simulink library "powerlib11"  (Simulink 6.0)
settings: Solver=ode45  SolverMode=SingleTasking  StartTime=0.0  StopTime=10.0  RelTol=1e-3
libraries: powerlib2 x45
settings Model: Creator=barnard  LastModifiedBy=batserve  ExtModeAutoUpdateStatusClock=off
settings OptimizationCC: BooleanDataType=off
settings DebuggingCC: SolverPrmCheckMsg=none
settings HardwareCC: TargetUnknown=on

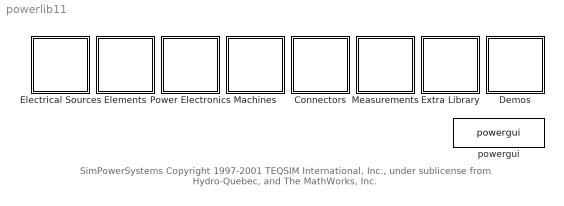
== system powerlib11 ==
  note: SimPowerSystems
      | Copyright  1997-2001 TEQSIM International, Inc., under sublicense
      | from Hydro-Quebec, and The MathWorks, Inc.
  Connectors : Subsystem
      mask Display: plot(0,0,100,100,[80,40],[40,40],[70,51],[31,31],[64,57],[23,23],[5,60,60],[70,70,40],[32,32],[70,97],[31,32,34,29,29,34,34,29,34,29],[71,68,71,71,70,68,71,68,68,71])
  Demos : Subsystem
      settings: OpenFcn=demo('simulink','SimPowerSystems')
      mask Display: disp('Demos')
  Electrical Sources : Subsystem
      mask Display: plot(-15,-15,15,15,[0 0 5 -5],[10 1.25 1.25 1.25],[0 0 -2 2],[-10 -1.25 -1.25 -1.25],[6 4 5 5 5]-10,[3 3 3 4 2]+3)
  Elements : Subsystem
      mask Display: plot(0,0,100,100,[90,64,77,77,60,56,51,46,40,34,30,25,13],[57,57,57,80,80,65,94,65,94,65,94,80,80],[90,87,82,77,74,68,64],[43,46,48,48,48,46,43],[48,77,77],[20,20,48],[39,27,13],[36,20,20])
  Extra Library : Subsystem
      settings: OpenFcn=powerlib_extras
      mask Display: disp('Extras')
  Machines : Subsystem
      mask Display: plot(-40,-40,40,40,[0,9,18,24,29,30,29,24,18,9,0,-9,-18,-24,-29,-30,-29,-24,-18,-9,0],[30,29,24,18,9,0,-9,-18,-24,-29,-30,-29,-24,-18,-9,0,9,18,24,29,30],[0,-9,-18,-24,-16,-16,-24,-18,-9,0,9,18,24,16,16,24,18,9,0]*.8,[-30,-29,-24,-18,-18,18,18,24,29,30,29,24,18,18,-18,-18,-24,-29,-30]*.8)
  Measurements : Subsystem  InitFcn=tag=strrep(tempname,tempdir,'');set_param(gcb,'VariableName',tag);
      mask Display: plot(-40,-40,40,60,[-30,-29,-24,-18,-9,0,9,18,24,29,30,-30],[0,9,18,24,29,30,29,24,18,9,0,0]*1.3,[0,10,3,10,12],[0,30,25,30,22])
  Power Electronics : Subsystem
      mask Display: plot(0,0,100,100,[50,30,70,50,30,70,50,50],[60,30,30,60,60,60,60,80],[50,50],[20,30],[30,41,44],[71,71,60])
  powergui : powerlib2/powergui  Frange=logspace(0,3,50)  Ylog=off  Xlog=off  save=off  variable=ZData  ZoomFFT=on  StartTime=0.0  cycles=2  DisplayStyle=off  fundamental=60  FreqAxis=off  MaxFrequency=1000  frequencyindice=1  frequencyindicesteady=1  RmsSteady=1  display=off  Ts=0  methode=off  frequency=60  echomessages=off

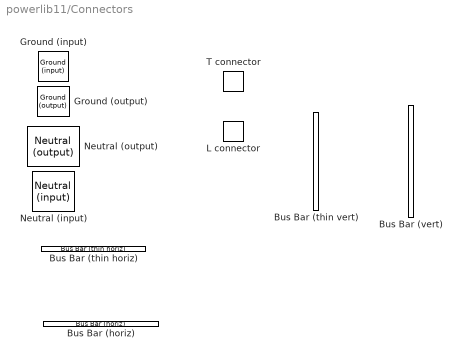
== system powerlib11/Connectors ==
  Bus Bar (horiz) : powerlib2/Connectors/Bus Bar (horiz)  Tag=PoWeRsYsTeMbLoCk  Orientation=down  entrees=2  sorties=1  PSBOutputType=1111111111111111111111111111111111111111111111111111111111111111111111111
  Bus Bar (thin horiz) : powerlib2/Connectors/Bus Bar (thin horiz)  Tag=PoWeRsYsTeMbLoCk  Orientation=down  input=2  output=1  PSBOutputType=111111111111111111111111111111111111111111111111111111111111111111111111111111111111
  Bus Bar (thin vert) : powerlib2/Connectors/Bus Bar (thin vert)  Tag=PoWeRsYsTeMbLoCk  input=2  output=1  PSBOutputType=111111111111111111111111111111111111111111111111111111111111111111111111111111111111
  Bus Bar (vert) : powerlib2/Connectors/Bus Bar (vert)  Tag=PoWeRsYsTeMbLoCk  entrees=3  sorties=2  PSBOutputType=11111111111111111111111111111111111111111111111111111111111111111111111111111111111111111
  Ground (input) : powerlib2/Connectors/Ground (input)  Tag=PoWeRsYsTeMbLoCk  Orientation=down
  Ground (output) : powerlib2/Connectors/Ground (output)  Tag=PoWeRsYsTeMbLoCk  Orientation=up  PSBOutputType=1
  L connector : powerlib2/Connectors/L connector  Tag=PoWeRsYsTeMbLoCk
  Neutral (input) : powerlib2/Connectors/Neutral (input)  Tag=PoWeRsYsTeMbLoCk  Orientation=down  no=99
  Neutral (output) : powerlib2/Connectors/Neutral (output)  Tag=PoWeRsYsTeMbLoCk  Orientation=up  no=99  PSBOutputType=1
  T connector : powerlib2/Connectors/T connector  Tag=PoWeRsYsTeMbLoCk  PSBOutputType=1

== system powerlib11/Demos ==

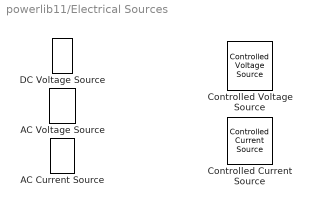
== system powerlib11/Electrical Sources ==
  AC Current Source : powerlib2/Electrical Sources/AC Current Source  Tag=PoWeRsYsTeMbLoCk  Description=source block  Orientation=up  A=10  P=0  F=60  stime=0  mesure=None  PSBOutputType=1
  AC Voltage Source : powerlib2/Electrical Sources/AC Voltage Source  Tag=PoWeRsYsTeMbLoCk  Description=source block  Orientation=up  A=100  P=0  F=60  stime=0  mesure=None  PSBOutputType=1
  Controlled Current Source : powerlib2/Electrical Sources/Controlled Current Source  Tag=PoWeRsYsTeMbLoCk  Description=source block  initsrc=on  srctyp=AC  ia=10  iph=0  freq=0  mesure=None  PSBOutputType=11
  Controlled Voltage Source : powerlib2/Electrical Sources/Controlled Voltage Source  Tag=PoWeRsYsTeMbLoCk  Description=source block  initsrc=on  srctyp=AC  iv=100  iph=0  ifreq=0  mesure=None  PSBOutputType=11
  DC Voltage Source : powerlib2/Electrical Sources/DC Voltage Source  Tag=PoWeRsYsTeMbLoCk  Description=source block  Orientation=up  V=100  mesure=None  PSBOutputType=1

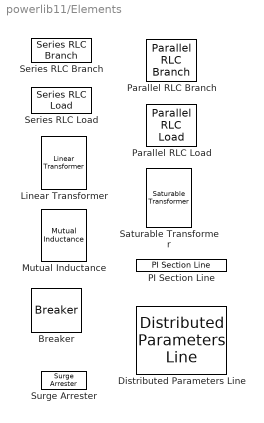
== system powerlib11/Elements ==
  Breaker : powerlib2/Elements/Breaker  Tag=PoWeRsYsTeMbLoCk  a=0.01  c=0  rs=inf  cs=0  times="[ 4/60  5/60 ]"  Ts=0  comext=on  mesure=None  PSBOutputType=1
  Distributed Parameters Line : powerlib2/Elements/Distributed Parameters Line  Tag=PoWeRsYsTeMbLoCk  n=3  f=60  r=[0.01273 0.3864]  l="[0.9337e-3  4.1264e-3]"  c=[12.74e-9 7.751e-9]  lgt=300  x1=[0 0 0 0; 0.0001244 0 0 0; 0.0002488 0 0 0; 0.0003733 0 0 0; 0.0004977 0 0 0; 0.0006221 0 0 0]  x2=[0 0 0 0; 0.0001244 0 0 0; 0.0002488 0 0 0; 0.0003733 0 0 0; 0.0004977 0 0 0; 0.0006221 0 0 0]  x3=[0 0 0 0; 0.0001244 0 0 0; 0.0002488 0 0 0; 0.0003733 0 0 0; 0.0004977 0 0 0; 0.0006221 0 0 0]  x4=[0 0 0 0; 0.0001244 0 0 0; 0.0002488 0 0 0; 0.0003733 0 0 0; 0.0004977 0 0 0; 0.0006221 0 0 0]  x5=0  mesure=None  PSBOutputType=111111111111111111111111111111
  Linear Transformer : powerlib2/Elements/Linear Transformer  Tag=PoWeRsYsTeMbLoCk  a=[250e6 60]  b=[735e3/sqrt(3) 0.002 0.08]  c=[315e3/sqrt(3) 0.002 0.08]  d=[60e3 0.005 0.02]  e=[500 500]  mesure=None  PSBOutputType=1111
  Mutual Inductance : powerlib2/Elements/Mutual Inductance  Tag=PoWeRsYsTeMbLoCk  a=[1.1 1.1e-03]  b=[ 1.1 1.1e-03]  c=[ 1.1 1.1e-03]  d=[1.0 1.0e-03]  mesure=None  PSBOutputType=111
  PI Section Line : powerlib2/Elements/PI Section Line  Tag=PoWeRsYsTeMbLoCk  f=60  a=0.2568  b=2e-03  c=8.6e-09  d=100  e=1  mesure=None  PSBOutputType=1
  Parallel RLC Branch : powerlib2/Elements/Parallel RLC Branch  Tag=PoWeRsYsTeMbLoCk  a=1  b=1e-03  c=1e-06  mesure=None  PSBOutputType=1
  Parallel RLC Load : powerlib2/Elements/Parallel RLC Load  Tag=PoWeRsYsTeMbLoCk  a=1000  b=60  c=10e3  d=100  e=100  mesure=None  PSBOutputType=1
  Saturable Transformer : powerlib2/Elements/Saturable Transformer  Tag=PoWeRsYsTeMbLoCk  a=[250e6 60]  b=[735e3/sqrt(3) 0.002 0.08]  c=[315e3/sqrt(3) 0.002 0.08]  d=[315e3/sqrt(3) 0.002 0.08]  e=[0 0 ; 0.001 1.2 ; 1 1.3]  f=[500]  H=off  matfile='hystXfo1'  Initialslope=+1  mesure=None  PSBOutputType=1111
  Series RLC Branch : powerlib2/Elements/Series RLC Branch  Tag=PoWeRsYsTeMbLoCk  a=1  b=1e-03  c=1e-06  mesure=None  PSBOutputType=1
  Series RLC Load : powerlib2/Elements/Series RLC Load  Tag=PoWeRsYsTeMbLoCk  a=1000  b=60  c=10e3  d=100  e=100  mesure=None  PSBOutputType=1
  Surge Arrester : powerlib2/Elements/Surge Arrester  Tag=PoWeRsYsTeMbLoCk  x1=500e+03  x2=2  x3=500  x4=[.955 50]  x5=[1.0 25]  x6=[.9915 16.5]  mesure=None  PSBOutputType=1

== system powerlib11/Extra Library ==

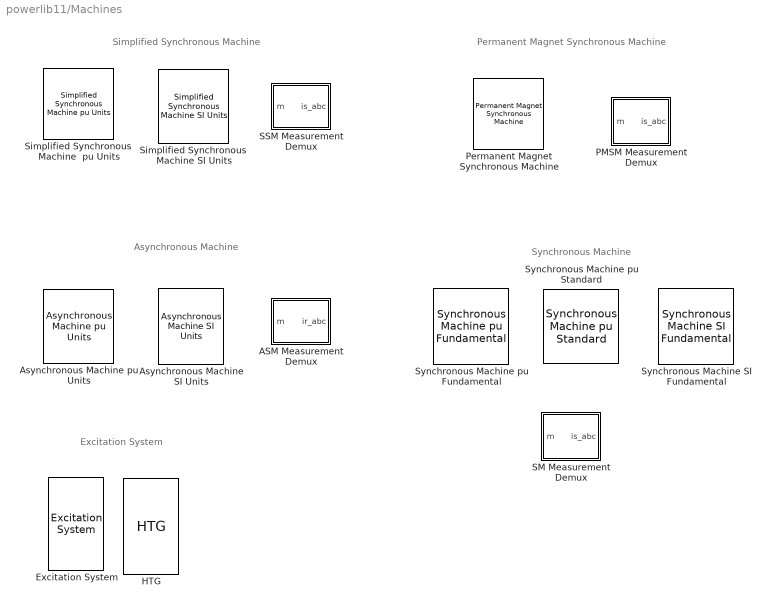
== system powerlib11/Machines ==
  note: Synchronous Machine
  note: Simplified Synchronous Machine
  note: Asynchronous Machine
  note: Permanent Magnet Synchronous Machine
  note: Excitation System
  ASM Measurement Demux : Subsystem  mask(Asynchronous Machine measurements){a=on, b=off, c=off, d=off, e=off, f=off, g=off, h=off, i=off, j=off, k=off}
      mask prompts: a "ir_abc       : Rotor currents ira, irb, irc (A) or (pu)"; b "ir_qd         : q and d axis rotor currents (A) or (pu)"; c "phir_qd    : q and d axis rotor fluxes (Wb) or (pu)"; d "vr_qd        : q and d axis rotor voltages (V) or (pu)"; e "is_abc      : Stator currents ia, ib, ic (A) or (pu)"; f "is_qd        : q and d axis stator currents (A) or (pu)"; g "phis_qd   : q and d axis stator fluxes (Wb) or (pu)"; h "vs_qd       : q and d axis stator voltages (V) or (pu)"; i "wm            : Rotor speed (rad/s) or (pu)"; j "Te              : Electromagnetic torque (N.m) or (pu)"; k "thetam      : Rotor angle (rad)"
      mask help: Split specified signals of Asynchronous Machine measurement output vector into separate signals. All electrical rotor quantities are referred to the stator.
      mask init:
      | bloc=gcb;
      | if strcmp(bdroot,'powerlib');return;end;
      | names={'ir_abc','ir_qd','phir_qd','vr_qd','is_abc','is_qd','phis_qd','vs_qd','wm','Te','thetam'};
      | etats={a,b,c,d,e,f,g,h,i,j,k};
      | OutNo = 0;
      | for i=1:11
      |    if etats{i}==0
      |       status='Terminator';
      |    else
      |       status='Outport';
      | 	  OutNo = OutNo+1;
      |    end
      |    actuel=get_param([bloc,'/',names{i}],'BlockType');
      |    if strcmp(actuel,status)==0
      |       replace_block(bloc,'FollowLinks','on','Name',names{i},status,'noprompt');
      | 	  if etats{i}==1
      | 	   set_param([bloc,'/',names{i}],'Port',num2str(OutNo));
      |        end
      |    end
      | end
  Asynchronous Machine SI Units : powerlib2/Machines/Asynchronous Machine SI Units  Tag=PoWeRsYsTeMbLoCk  rotType=Wound  ctrl=Rotor  x1=[ 3*746, 220, 60 ]  x2="[ 0.435  2.0e-3 ]"  x3="[ 0.816  2.0e-3 ]"  x4=69.31e-3  x5="[ 0.089  0  2 ]"  x6="[ 1,0   0,0,0   0,0,0 ]"  PSBOutputType=1110  iounits=1
  Asynchronous Machine pu Units : powerlib2/Machines/Asynchronous Machine pu Units  Tag=PoWeRsYsTeMbLoCk  rotType=Wound  ctrl=Rotor  x1=[ 3*746, 220, 60 ]  x2=[ 0.0201,0.0349 ]  x3=[ 0.0377,0.0349 ]  x4=1.2082  x5=[ 0.7065,0,2 ]  x6="[ 1,0   0,0,0   0,0,0 ]"  PSBOutputType=1110  iounits=0
  Excitation System : powerlib2/Machines/Excitation System  tr=20e-3  reg=[ 300, 0.001 ]  exc=[ 1, 0 ]  tgr=[ 0, 0 ]  damp=[ 0.001, 0.1 ]  sat=[ 0, 0 ]  lim=[ -11.5, 11.5, 0 ]  v0="[1.0  1.28]"
  HTG : powerlib2/Machines/HTG  sm="[ 10/3  0.07 ]"  gate="[  0.01  0.97518  -0.1  0.1 ]"  reg="[  0.05  1.163  0.105  0  0.01  ]"  hyd="[  0  2.67  ]"  dref=0  po=0.7516
  PMSM Measurement Demux : Subsystem  mask(Permanent Magnet Synchronous Machine measurements){a=on, b=off, c=off, d=off, e=off, f=off}
      mask prompts: a "is_abc  : Stator line currents ia, ib, ic (A)"; b "is_qd    : q and d axis stator currents (A)"; c "vs_qd   : q and d axis stator voltages (V)"; d "wm        : Rotor speed (rad/s)"; e "thetam  : Rotor angle (rad)"; f "Te          : Electromagnetic torque (N.m)"
      mask help: Split specified signals of Permanent Magnet Synchronous Machine measurement output vector into separate signals.
      mask init:
      | bloc=gcb;
      | if strcmp(bdroot,'powerlib');return;end
      | names={'is_abc','is_qd','vs_qd','wm','thetam','Te'};
      | etats={a,b,c,d,e,f};
      | OutNo = 0;
      | for i=1:6
      |    if etats{i}==0
      |       status='Terminator';
      |    else
      |       status='Outport';
      | 	  OutNo = OutNo+1;
      |    end
      |    actuel=get_param([bloc,'/',names{i}],'BlockType');
      |    if strcmp(actuel,status)==0
      |       replace_block(bloc,'FollowLinks','on','Name',names{i},status,'noprompt');
      | 	  if etats{i}==1
      | 	  set_param([bloc,'/',names{i}],'Port',num2str(OutNo));
      |       end
      |    end
      | end
  Permanent Magnet Synchronous Machine : powerlib2/Machines/Permanent Magnet Synchronous Machine  Tag=PoWeRsYsTeMbLoCk  x1=2.875  x2=[8.5e-3, 8.5e-3]  x3=0.175  x4="[ 0.8e-3, 0,  4 ]"  PSBOutputType=0
  SM Measurement Demux : Subsystem  mask(Synchronous Machine measurements){a=on, b=off, c=off, d=off, e=off, f=off, g=off, h=off, i=off, j=off}
      mask prompts: a "is_abc      : Stator currents isa, isb, isc (A) or (pu)"; b "is_qd        : q and d axis stator currents (A) or (pu)"; c "ifd              : Field current (A) or (pu)"; d "ik_qd        : Damper winding currents ikq1, ikq2, ikd (A) or (pu)"; e "phim_qd  : q and d axis mutual fluxes"; f "vs_qd       : q and d axis stator voltages (V) or (pu)"; g "theta        : Rotor mechanical angle (deg)"; h "wm            : Rotor speed (rad/s) or (pu)"; i "Pe             : Electrical power (W) or (pu)"; j "dw             : Rotor speed deviation (pu)"
      mask help: Split specified signals of Synchronous Machine measurement output vector into separate signals. Damper winding currents are referred to the stator.
      mask init:
      | bloc=gcb;
      | if strcmp(bdroot,'powerlib');return;end;
      | names={'is_abc','is_qd','ifd','ik_qd','phim_qd','vs_qd','theta','wm','Pe','dw'};
      | etats={a,b,c,d,e,f,g,h,i,j};
      | OutNo = 0;
      | for i=1:10
      |    if etats{i}==0
      |       status='Terminator';
      |    else
      |       status='Outport';
      |       OutNo = OutNo+1;
      |    end
      |    actuel=get_param([bloc,'/',names{i}],'BlockType');
      |    if strcmp(actuel,status)==0
      | 	   replace_block(bloc,'FollowLinks','on','Name',names{i},status,'noprompt');
      | 	   if etats{i}==1
      | 	   set_param([bloc,'/',names{i}],'Port',num2str(OutNo));
      |        end
      |    end
      | end
  SSM Measurement Demux : Subsystem  mask(Simplified Synchronous Machine measurements){a=on, b=off, c=off, d=off, e=off, f=off}
      mask prompts: a "is_abc  : Line currents ia, ib, ic (A) or (pu)"; b "vs_abc : Terminal voltages va, vb, vc (V) or (pu)"; c "e_abc   : Internal voltages ea, eb, ec (V) or (pu)"; d "thetam  : Rotor angle (rad)"; e "wm        : Rotor speed (rad/s) or (pu)"; f "Pe         : Electrical power (W)  or  (pu)"
      mask help: Split specified signals of Simplified Synchronous Machine measurement output vector into separate signals.
      mask init:
      | bloc=gcb;
      | if strcmp(bdroot,'powerlib');return;end
      | names={'is_abc','vs_abc','e_abc','thetam','wm','Pe'};
      | etats={a,b,c,d,e,f};
      | OutNo = 0;
      | for i=1:6
      |    if etats{i}==0
      |       status='Terminator';
      |    else
      |       status='Outport';
      | 	  OutNo = OutNo+1;
      |    end
      |    actuel=get_param([bloc,'/',names{i}],'BlockType');
      |    if strcmp(actuel,status)==0
      |       replace_block(bloc,'FollowLinks','on','Name',names{i},status,'noprompt');
      | 	  if etats{i}==1
      | 	   set_param([bloc,'/',names{i}],'Port',num2str(OutNo));
      |        end
      |    end
      | end
  Simplified Synchronous  Machine  pu Units : powerlib2/Machines/Simplified Synchronous  Machine  pu Units  Tag=PoWeRsYsTeMbLoCk  conType=3-wire Y  x1=[ 1000e6,315e3,60 ]  x2=[ inf,0,2 ]  x3=[ 0.02,1 ]  x4="[ 0   0   0,0,0   0,0,0 ]"  PSBOutputType=1110  iounits=0
  Simplified Synchronous  Machine SI Units : powerlib2/Machines/Simplified Synchronous  Machine SI Units  Tag=PoWeRsYsTeMbLoCk  conType=3-wire Y  x1=[ 1000e6,315e3,60 ]  x2=[ inf,0,2 ]  x3=[ 1.9845,263.15e-3 ]  x4="[ 0   0   0,0,0   0,0,0 ]"  PSBOutputType=1110  iounits=1
  Synchronous Machine SI Fundamental : powerlib2/Machines/Synchronous Machine SI Fundamental  Tag=PoWeRsYsTeMbLoCk  rotorType=Salient-pole  x1="[ 187E6  13800   60   1087 ]"  x2="[ 2.9069E-03  3.0892E-04  3.2164E-03  9.7153E-04 ]"  x3="[ 5.9013E-04  3.0712E-04 ]"  x4b=[ 0.0664, 1.387e-3, 0.0292, 6.896e-4, 7.907e-3, 2.477e-3]  x4="[ 1.1900E-02  4.9076E-04  2.0081E-02  1.0365E-03 ]"  x5="[ inf  0  20 ]"  x6="[ 0  0  0  0  0  0  0  0  70.3192 ]"  x7=off  x8=[695.64,774.7,917.5,1001.6,1082.2,1175.9,1293.6,1430.2,1583.7;9660,10623,12243,13063,13757,14437,15180,15890,16567]  x9=off  PSBOutputType=1110  iounits=1
  Synchronous Machine pu Fundamental : powerlib2/Machines/Synchronous Machine pu Fundamental  Tag=PoWeRsYsTeMbLoCk  rotorType=Salient-pole  x1="[ 187E6  13800   60 ]"  x2="[ 2.8544E-03  0.11436  1.1906  0.35964 ]"  x3="[ 5.7947E-04  0.11369 ]"  x4b=[0.0652, 0.5134, 0.0287, 0.2553, 7.765e-3, 0.9167 ]  x4="[ 1.1685E-02  0.18167  1.9718E-02  038371 ]"  x5="[ inf  0  20 ]"  x6="[ 0  0  0  0  0  0  0  0  1 ]"  x7=off  x8=[0.6404,0.7127,0.8441,0.9214,0.9956,1.082,1.19,1.316,1.457;0.7,0.7698,0.8872,0.9466,0.9969,1.046,1.1,1.151,1.201]  PSBOutputType=1110  iounits=0
  Synchronous Machine pu Standard : powerlib2/Machines/Synchronous Machine pu Standard  Tag=PoWeRsYsTeMbLoCk  rotorType=Salient-pole  x1="[ 187E6  13800   60 ]"  x2b=[ 1.81, 0.3, 0.23, 1.76, 0.65, 0.25, 0.15 ]  x2=[ 1.305, 0.296, 0.252, 0.474, 0.243, 0.18 ]  dAxisT=Open-circuit  qAxisT=Short-circuit  x3a="[ 4.4849  0.0681  0.1  ]"  x3b=[ 8.0, 0.03, 1.0, 0.07 ]  x3c="[  4.4849  0.0681  0.051266  ]"  x3d=[ 8.0, 0.03, 0.3371, 0.0295 ]  x3=[ 1.01, 0.053, 0.1 ]  x3e=[ 1.3201, 0.023, 1.0, 0.07 ]  x3f="[  1.01  0.053  0.051266  ]"  x3g=[ 1.3201, 0.0231, 0.3371, 0.0295 ]  x4=0.003  x5="[ inf  0  20 ]"  x6="[ 0  0  0  0  0  0  0  0  1 ]"  x7=off  x8=[0.6404,0.7127,0.8441,0.9214,0.9956,1.082,1.19,1.316,1.457;0.7,0.7698,0.8872,0.9466,0.9969,1.046,1.1,1.151,1.201]  PSBOutputType=1110  iounits=0.5

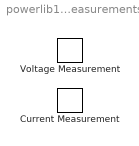
== system powerlib11/Measurements ==
  Current Measurement : powerlib2/Measurements/Current Measurement  Tag=PoWeRsYsTeMmEaSuReMeNt  PSBOutputType=01  PSBequivalent=0
  Voltage Measurement : powerlib2/Measurements/Voltage Measurement  Tag=PoWeRsYsTeMmEaSuReMeNt  PSBOutputType=0  PSBequivalent=0

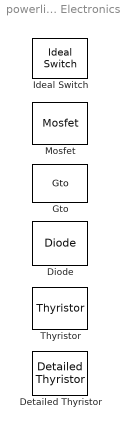
== system powerlib11/Power Electronics ==
  Detailed Thyristor : powerlib2/Power Electronics/Detailed Thyristor  Tag=PoWeRsYsTeMbLoCk  Ron=1e-3  Lon=0  Vf=0.8  IL=0.1  Tq=100e-6  IC=0  Rs=10  Cs=4.7e-6  PSBOutputType=10
  Diode : powerlib2/Power Electronics/Diode  Tag=PoWeRsYsTeMbLoCk  Ron=0.01  Lon=0  Vf=0.8  IC=0  Rs=10  Cs=0.01e-6  PSBOutputType=10
  Gto : powerlib2/Power Electronics/Gto  Tag=PoWeRsYsTeMbLoCk  Ron=0.01  Lon=1e-6  Vf=1  Tf=10e-6  Tt=20e-6  IC=0  Rs=10  Cs=0.01e-6  PSBOutputType=10
  Ideal Switch : powerlib2/Power Electronics/Ideal Switch  Tag=PoWeRsYsTeMbLoCk  Ron=0.01  Lon=0  IC=0  Rs=10  Cs=0.01e-6  PSBOutputType=10
  Mosfet : powerlib2/Power Electronics/Mosfet  Tag=PoWeRsYsTeMbLoCk  Ron=0.001  Lon=1e-6  Rd=.001  IC=0  Rs=10  Cs=0.01e-6  PSBOutputType=10
  Thyristor : powerlib2/Power Electronics/Thyristor  Tag=PoWeRsYsTeMbLoCk  Ron=1e-03  Lon=0  Vf=0.8  IC=0  Rs=10  Cs=4.7e-6  PSBOutputType=10

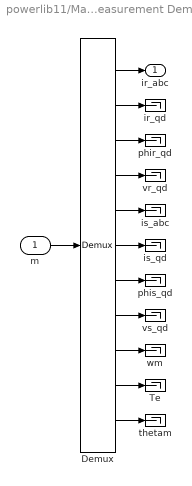
== system powerlib11/Machines/ASM Measurement Demux ==
  m : Inport  Port=1  LatchInput=off
  Demux : Demux  Outputs=[3,2,2,2,3,2,2,2,1,1,1]
  Te : Terminator
  ir_qd : Terminator
  is_abc : Terminator
  is_qd : Terminator
  phir_qd : Terminator
  phis_qd : Terminator
  thetam : Terminator
  vr_qd : Terminator
  vs_qd : Terminator
  wm : Terminator
  ir_abc : Outport
  wires:
  m/1 -> Demux/1
  Demux/1 -> ir_abc/1
  Demux/2 -> ir_qd/1
  Demux/3 -> phir_qd/1
  Demux/4 -> vr_qd/1
  Demux/5 -> is_abc/1
  Demux/6 -> is_qd/1
  Demux/7 -> phis_qd/1
  Demux/8 -> vs_qd/1
  Demux/9 -> wm/1
  Demux/10 -> Te/1
  Demux/11 -> thetam/1

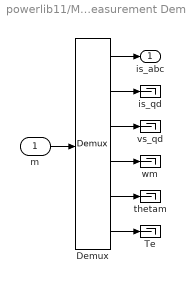
== system powerlib11/Machines/PMSM Measurement Demux ==
  m : Inport  Port=1  LatchInput=off
  Demux : Demux  Outputs=[3,2,2,1,1,1]
  Te : Terminator
  is_qd : Terminator
  thetam : Terminator
  vs_qd : Terminator
  wm : Terminator
  is_abc : Outport
  wires:
  m/1 -> Demux/1
  Demux/1 -> is_abc/1
  Demux/2 -> is_qd/1
  Demux/3 -> vs_qd/1
  Demux/4 -> wm/1
  Demux/5 -> thetam/1
  Demux/6 -> Te/1

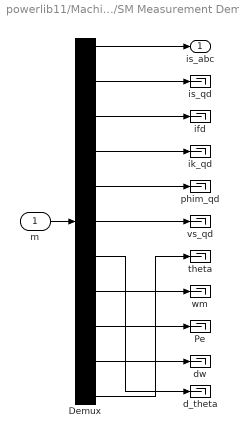
== system powerlib11/Machines/SM Measurement Demux ==
  m : Inport  Port=1  LatchInput=off
  Demux : Demux  Outputs=[3,2,1,3,2,2,1,1,1,1,1]
  Pe : Terminator
  d_theta : Terminator
  dw : Terminator
  ifd : Terminator
  ik_qd : Terminator
  is_qd : Terminator
  phim_qd : Terminator
  theta : Terminator
  vs_qd : Terminator
  wm : Terminator
  is_abc : Outport
  wires:
  m/1 -> Demux/1
  Demux/1 -> is_abc/1
  Demux/2 -> is_qd/1
  Demux/3 -> ifd/1
  Demux/4 -> ik_qd/1
  Demux/5 -> phim_qd/1
  Demux/6 -> vs_qd/1
  Demux/8 -> wm/1
  Demux/9 -> Pe/1
  Demux/10 -> dw/1
  Demux/11 -> theta/1
  Demux/7 -> d_theta/1

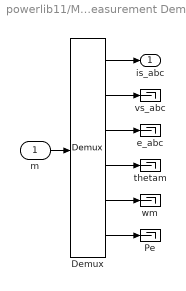
== system powerlib11/Machines/SSM Measurement Demux ==
  m : Inport  Port=1  LatchInput=off
  Demux : Demux  Outputs=[3,3,3,1,1,1]
  Pe : Terminator
  e_abc : Terminator
  thetam : Terminator
  vs_abc : Terminator
  wm : Terminator
  is_abc : Outport
  wires:
  Demux/6 -> Pe/1
  Demux/5 -> wm/1
  Demux/4 -> thetam/1
  Demux/3 -> e_abc/1
  Demux/2 -> vs_abc/1
  Demux/1 -> is_abc/1
  m/1 -> Demux/1
